simulink model "pp_c_ss"  (Simulink 5.0)
settings: Solver=ode23s  StartTime=t0  StopTime=tf  RelTol=1e-8  AbsTol=1.0e-8
values from neighbouring files (symbols this model uses):
  a = [0 0;1 -0.1]    [ant.m]    (also in motor.m = [-1 0; 1 0]; sigurd.m = 0.9)
  b = [0.1; 0]    [ant.m]    (also in motor.m = [1; 0])
  c = [0 1]    [ant.m]    (also in motor.m)
  d = 0    [ant.m]    (also in motor.m)
  R = 9.76e-4*[1 -0.5625]    [pplace2.m]
  S = 0.1426    [pplace2.m]
  st = 1    [ant.m]    (also in dof_choice.m; motor.m; roll_im.m = 0.2; sigurd.m)
  Ts = 0.2; [B,A,k] = myc2d(G,Ts)    [ant.m]    (also in dof_choice.m = 1; motor.m = 0.25; [B,A,k] = myc2d(G,Ts); roll_im.m = 0.001; sigurd.m = 0.025)
  xInitial = [0 0]    [ant.m]    (also in dof_choice.m; motor.m; roll_im.m = [0 0.2 0 0 0 0 0]; type_2DOF.m)
undefined symbols (not defined in the file or in its folder): TM
settings Model: Creator=kannanm  LastModifiedBy=kannan  ExtModeAutoUpdateStatusClock=off  SaveState=on  StateSaveName=xinit

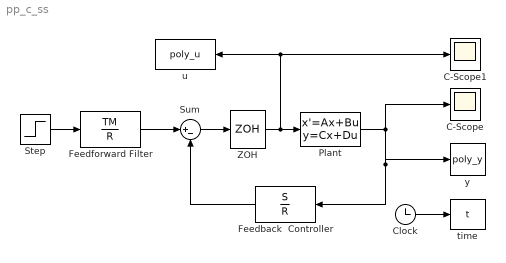
== system pp_c_ss ==
  C-Scope : Scope
      settings: YMin=0  YMax=1.2
  C-Scope1 : Scope
      settings: YMin=0  YMax=1.2
  Clock : Clock
      settings: Decimation=10
  Feedback  Controller : DiscreteFilter  Orientation=left  Numerator=S  Denominator=R  SampleTime=Ts
  Feedforward Filter : DiscreteFilter  Numerator=TM  Denominator=R  SampleTime=Ts
  Plant : StateSpace  A=a  B=b  C=c  D=d  X0=xInitial
  Step : Step  Time=0  After=st  SampleTime=Ts
  Sum : Sum  Inputs=|+-  SaturateOnIntegerOverflow=on
  ZOH : ZeroOrderHold  SampleTime=Ts
  time : ToWorkspace  VariableName=t  SampleTime=Ts  SaveFormat=Array
  u : ToWorkspace  VariableName=poly_u  SampleTime=Ts  SaveFormat=Array
  y : ToWorkspace  VariableName=poly_y  SampleTime=Ts  SaveFormat=Array
  wires:
  Step/1 -> Feedforward Filter/1
  Feedforward Filter/1 -> Sum/1
  Sum/1 -> ZOH/1
  Feedback  Controller/1 -> Sum/2
  ZOH/1 -> Plant/1, u/1, C-Scope1/1
  Clock/1 -> time/1
  Plant/1 -> Feedback  Controller/1, y/1, C-Scope/1
